simulink model "PartB1"  (R2025b)
settings: Solver=VariableStepAuto  StartTime=0.0  StopTime=10.0  RelTol=1e-3
settings Model: Creator=safiakhalil  LastModifiedBy=safiakhalil

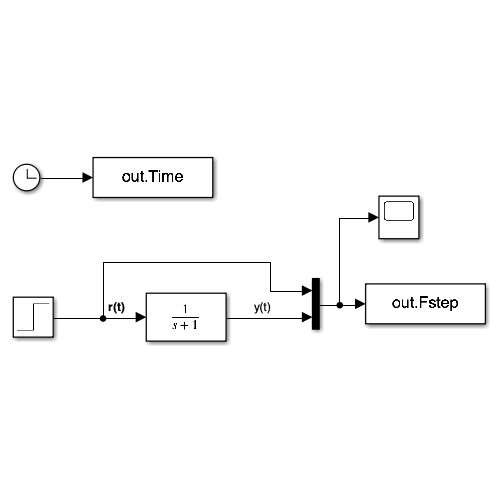
[thumbnail: Simulink's stored preview of the top-level diagram]
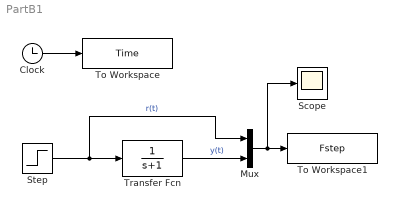
== system PartB1 ==
  Clock : Clock
  Mux : Mux  Inputs=2
  Scope : Scope
      settings: ActiveDisplayYMinimum=0.59802018633540377  ActiveDisplayYMaximum=0.65236801242236031  YLabel=Y-axis
  Step : Step  SampleTime=0
  To Workspace : ToWorkspace  VariableName=Time  SampleTime=-1
  To Workspace1 : ToWorkspace  VariableName=Fstep  SampleTime=-1
  Transfer Fcn : TransferFcn  Denominator=[1 1]
  wires:
  Clock/1 -> To Workspace/1
  Step/1 -> Mux/1, Transfer Fcn/1  "r(t)"
  Transfer Fcn/1 -> Mux/2  "y(t)"
  Mux/1 -> To Workspace1/1, Scope/1
